simulink model "drilling_openloop_sim"  (R2024b)
settings: Solver=ode4  StartTime=0.0  StopTime=75*60  FixedStep=0.1  RelTol=1e-3
libraries: realtime_pacer_lib x1
settings Model: PacingRate=60  Creator=Torstein  LastModifiedBy=Torstein

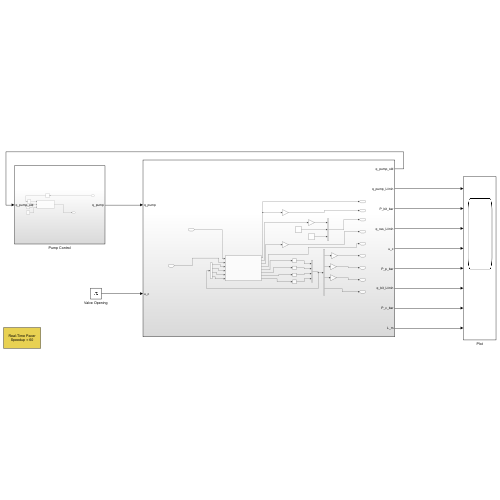
[thumbnail: Simulink's stored preview of the top-level diagram]
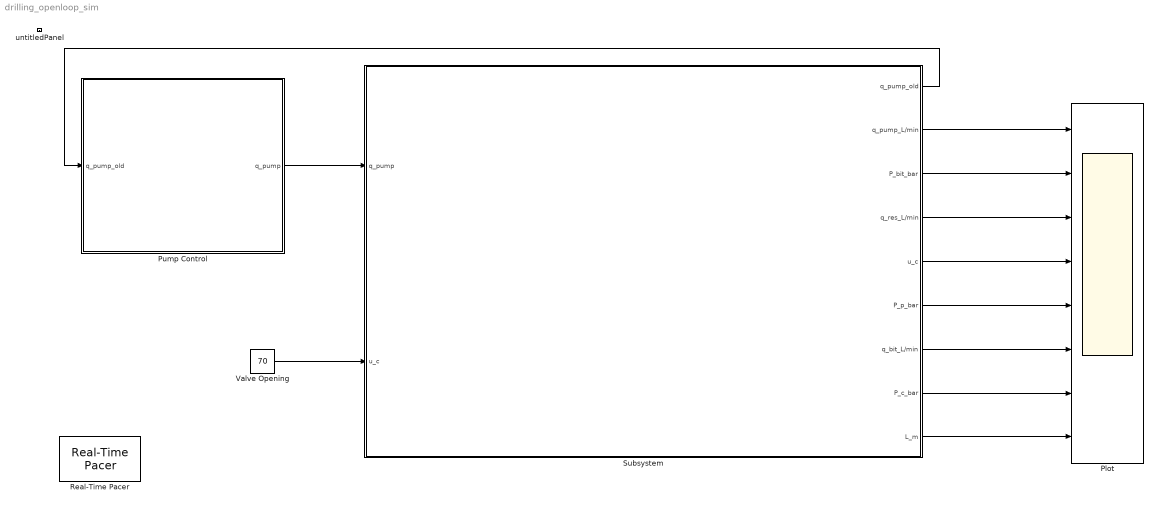
== system drilling_openloop_sim ==
  Plot : Scope  NumInputPorts=8
  Pump Control : Subsystem
  Real-Time Pacer : realtime_pacer_lib/Real-Time Pacer  simTimePerRealTime=60
      settings: SourceProductName=Real-Time Pacer
  Subsystem : Subsystem
  Valve Opening : Constant  Value=70
  untitledPanel : Subsystem  Tag=HiddenForWebPanel  IsWebBlockPanel=on
  wires:
  Pump Control/1(q_pump) -> Subsystem/1("q_pump ")
  Valve Opening/1 -> Subsystem/2("u_c ")
  Subsystem/4(q_res_L/min) -> Plot/3
  Subsystem/5(u_c) -> Plot/4
  Subsystem/6(P_p_bar) -> Plot/5
  Subsystem/7(q_bit_L/min) -> Plot/6
  Subsystem/8(P_c_bar) -> Plot/7
  Subsystem/9(L_m) -> Plot/8
  Subsystem/3(P_bit_bar) -> Plot/2
  Subsystem/2(q_pump_L/min) -> Plot/1
  Subsystem/1(q_pump_old) -> Pump Control/1(q_pump_old)

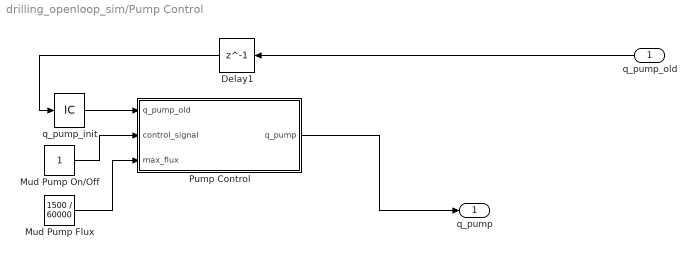
== system drilling_openloop_sim/Pump Control ==
  q_pump_old : Inport
  Delay1 : Delay  DelayLength=1  InitialCondition=0
  Mud Pump Flux : Constant  Value=1500 / 60000
  Mud Pump On/Off : Constant
  Pump Control : MATLAB Function  TreatAsAtomicUnit=on
  q_pump_init : InitialCondition  Value=1500 / 60000
  q_pump : Outport
  wires:
  q_pump_old/1 -> Delay1/1
  Delay1/1 -> q_pump_init/1
  Mud Pump Flux/1 -> Pump Control/3(max_flux)
  Mud Pump On/Off/1 -> Pump Control/2(control_signal)
  Pump Control/1(q_pump) -> q_pump/1
  q_pump_init/1 -> Pump Control/1(q_pump_old)

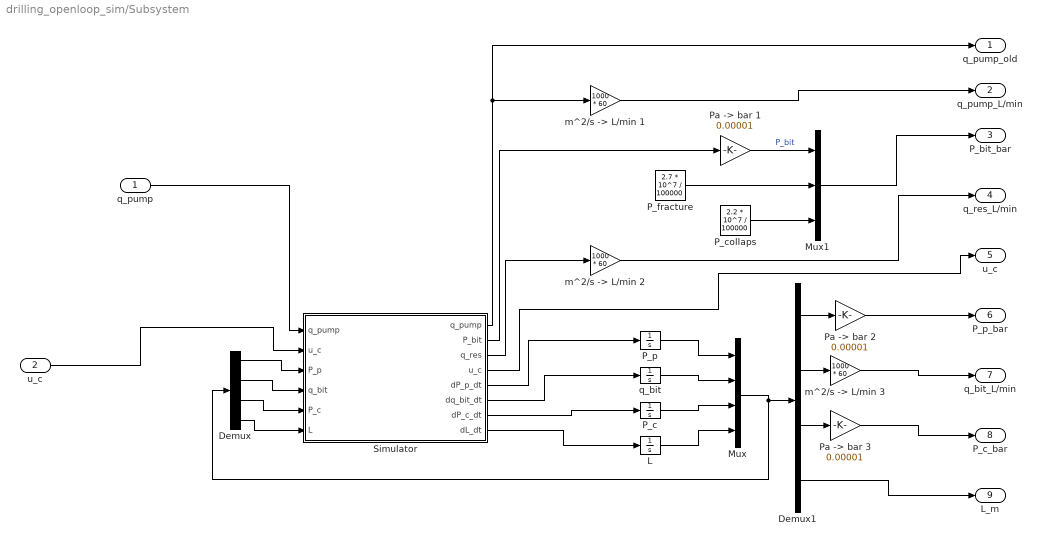
== system drilling_openloop_sim/Subsystem ==
  "q_pump " : Inport
  "u_c " : Inport  Port=2
  Demux : Demux
  Demux1 : Demux
  L : Integrator  InitialCondition=1600
  Mux : Mux
  Mux1 : Mux  Inputs=3
  P_c : Integrator  InitialCondition=5.5 * 10^6
  P_collaps : Constant  Value=2.2 * 10^7 / 100000
  P_fracture : Constant  Value=2.7 * 10^7 / 100000
  P_p : Integrator  InitialCondition=5 * 10^6
  "Pa -> bar 1" : Gain  Gain=0.00001
  "Pa -> bar 2" : Gain  Gain=0.00001
  "Pa -> bar 3" : Gain  Gain=0.00001
  Simulator : MATLAB Function  TreatAsAtomicUnit=on
  "m^2/s -> L/min 1" : Gain  Gain=1000 * 60
  "m^2/s -> L/min 2" : Gain  Gain=1000 * 60
  "m^2/s -> L/min 3" : Gain  Gain=1000 * 60
  q_bit : Integrator  InitialCondition=0.025
  q_pump_old : Outport
  q_pump_L/min : Outport  Port=2
  P_bit_bar : Outport  Port=3
  q_res_L/min : Outport  Port=4
  u_c : Outport  Port=5
  P_p_bar : Outport  Port=6
  q_bit_L/min : Outport  Port=7
  P_c_bar : Outport  Port=8
  L_m : Outport  Port=9
  wires:
  Demux/2 -> Simulator/4(q_bit)
  Demux/1 -> Simulator/3(P_p)
  Simulator/2(P_bit) -> "Pa -> bar 1"/1
  Simulator/6(dq_bit_dt) -> q_bit/1
  Simulator/3(q_res) -> "m^2/s -> L/min 2"/1
  "m^2/s -> L/min 2"/1 -> q_res_L/min/1
  Demux1/3 -> "Pa -> bar 3"/1
  Demux1/1 -> "Pa -> bar 2"/1
  P_fracture/1 -> Mux1/2
  Simulator/1(q_pump) -> q_pump_old/1, "m^2/s -> L/min 1"/1
  Simulator/5(dP_p_dt) -> P_p/1
  L/1 -> Mux/4
  Mux/1 -> Demux1/1, Demux/1
  Demux1/4 -> L_m/1
  P_c/1 -> Mux/3
  "Pa -> bar 2"/1 -> P_p_bar/1
  q_bit/1 -> Mux/2
  Simulator/8(dL_dt) -> L/1
  Demux/3 -> Simulator/5(P_c)
  P_collaps/1 -> Mux1/3
  "Pa -> bar 1"/1 -> Mux1/1  "P_bit"
  Demux1/2 -> "m^2/s -> L/min 3"/1
  P_p/1 -> Mux/1
  Simulator/7(dP_c_dt) -> P_c/1
  Demux/4 -> Simulator/6(L)
  Simulator/4(u_c) -> u_c/1
  "Pa -> bar 3"/1 -> P_c_bar/1
  "m^2/s -> L/min 3"/1 -> q_bit_L/min/1
  "u_c "/1 -> Simulator/2("u_c ")
  "q_pump "/1 -> Simulator/1("q_pump ")
  Mux1/1 -> P_bit_bar/1
  "m^2/s -> L/min 1"/1 -> q_pump_L/min/1

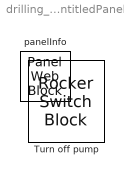
== system drilling_openloop_sim/untitledPanel ==
  Turn off pump : RockerSwitchBlock  Tag=HiddenForWebPanel  PanelInfo="{\"height\":82,\"left\":22,\"panelId\":\"panelId-269a8be7-2ea9-4a07-85fb-b2e5eec89753\",\"top\":21,\"type\":\"panelChild\",\"version\":\"2019b\",\"width\":76,\"zIndex\":1500002}"
      settings: Values={{'Off', 'On'}, [-1 1]}
  panelInfo : PanelWebBlock  Tag=HiddenForWebPanel  PanelInfo="{\"compacted\":false,\"height\":122,\"isActiveTab\":true,\"left\":503,\"name\":\"Panel\",\"panelId\":\"panelId-269a8be7-2ea9-4a07-85fb-b2e5eec89753\",\"tabIndex\":0,\"tabbedSetId\":\"tabbedSet3531040432\",\"top\":33,\"type\":\"panel\",\"version\":\"2019b\",\"visible\":true,\"width\":116,\"zIndex\":1500002}"

== matlab function drilling_openloop_sim/Subsystem/Simulator ==
  data: q_pump output; P_bit output; q_res output; u_c output; q_pump input; dP_p_dt output; u_c input; P_p input; q_bit input; dq_bit_dt output; dP_c_dt output; dL_dt output; P_c input; L input
function [q_pump, P_bit, q_res, u_c, dP_p_dt, dq_bit_dt, dP_c_dt, dL_dt] = Pressure_equation(q_pump, u_c, P_p, q_bit, P_c, L)
    % Initial conditions
    % P_p                               # Mud pump downstream pressure
    % q_bit                             # Volum flux of drill mud through drill bit
    % P_c                               # Well head pressure at annulus
    % L = (1600) m		                # Depth of well

    % Constants
    % u_c = (70) \%		                # Choke Valve opening
    % q_pump (0.025) m^3/s              # Volum flux of drill mud through mud pump
    beta_d = 3 * 10^8; % N/m^2	        # Bulk modulus at drill string
    A_d = 0.0067; % m^2                 # Area of drill string cross section
    g = 9.81; % m/s^2    		        # Gravitational acceleration
    beta_a = 2.4 * 10^8; % N/m^2	    # Bulk modulus at annulus
    A_a = 0.278; % m^2		            # Area of annulus cross section
    q_back = 0; % m^2/s			        # Volum flux of backpressure pump
    P_0 = 4 * 10^5; % N/m^2	            # Pressure downstream from choke valve
    rho_w = 1000; % kg/m^3	    	    # Water density
    W_c = 0.1; %    			        # Water cut/ratio in reservoir fluid
    rho_l = 1150; % kg/m^3		        # Density of drill mud
    P_i	= 1.6667 * 10^(-9); % m^5/Ns    # Productivity index of well
    P_res = 2.5 * 10^7; % N/m^2	        # Reservoir pressure
    v_pen = 0; % m/s	        		# Drilling speed
    D_hd = 0.0925; % m          	    # Hydraulic diameter of drill string
    D_ha = 0.211; % m          	        # Hydraulic diameter of annual

    % Parameters
    rho_mix = rho_w * W_c + (1 - W_c) * rho_l;

    %Z_c = max([0, 0.111 * u_c - 0.556, 0.5 * u_c - 20]);
    Z_c = calc_Z_c;

    q_choke = 27.3 / (3600 * sqrt(10^5)) * Z_c * sqrt(max([0, P_c - P_0]) / rho_mix);

    DeltaP_fd = calc_DeltaP_f(rho_l, q_pump, A_d, D_hd);
    DeltaP_fa = calc_DeltaP_f(rho_mix, q_choke, A_a, D_ha);

    P_bit = P_c + rho_mix * g * L + DeltaP_fa;

    q_res = max([0, P_i * (P_res - P_bit)]);


    % Differnetial equations
    dP_p_dt = beta_d / (A_d * L) * (q_pump - q_bit);

    if q_bit <= 0
        dq_bit_dt = max([0, A_d / (rho_l * L) * (P_p + rho_l * g * L - DeltaP_fd - P_bit)]);
    else
        dq_bit_dt = A_d / (rho_l * L) * (P_p + rho_l * g * L - DeltaP_fd - P_bit);
    end

    dP_c_dt = beta_a / (A_a * L) * (q_bit + q_res + q_back - q_choke);

    dL_dt = v_pen;

    % Functions
    function res = calc_Z_c
        if 0.111 * u_c - 0.556 < 0
            res = 0;
        elseif u_c < 50
            res = 0.111 * u_c - 0.556;
        else
            res = 0.5 * u_c - 20;
        end
    end

    function res = calc_DeltaP_f(rho_x, q_x, A_x, D_hx)
        f_d = 0.02; %        			# Friction factor.

        v_x = q_x / A_x;
        res = f_d * L * rho_x * v_x^2 / (2 * D_hx);
    end

end

== matlab function drilling_openloop_sim/Pump Control/Pump Control ==
  data: q_pump_old input; q_pump output; control_signal input; max_flux input
function q_pump = pump_spinner(q_pump_old, control_signal, max_flux)
    step = 30/60000 / 60;
    q_pump = q_pump_old;

    if control_signal > 0
        if q_pump_old < max_flux
            q_pump = q_pump_old + step;
        end
        if q_pump > max_flux
            q_pump = max_flux;
        end
    elseif control_signal <= 0
        if q_pump_old > 0
            q_pump = q_pump_old - step;
        end
        if q_pump < 0
            q_pump = 0.0;
        end
    end
end
